simulink model "LQR_discrete"  (R2022a)
settings: Solver=VariableStepAuto  StartTime=0.0  StopTime=T_sim  RelTol=1e-3
values from neighbouring files (symbols this model uses):
  A = [-1.2822  0      0.98     0 ... (first row only)    [main.m]    (also in main_cessna.m = [-1.2822 0 0.98 0)
  B = [-0.3 ... (first row only)    [main.m]    (also in main_cessna.m)
  C = [0       1      0  0 ... (first row only)    [main.m]    (also in main_cessna.m = [0 1 0 0)
  C_states = eye(length(A))    [main.m]    (also in main_cessna.m = eye(4))
  D_states = zeros(length(B), 1)    [main.m]
  k_LQ = k_LQ4    [main.m]
  sysd = c2d(sys,T_sampling)    [main.m]
  T_sampling = 2*pi/omega_sampling    [main.m]
  u_max = deg2rad(15)    [main.m]
  u_min = deg2rad(-15)    [main.m]
  x0 = [deg2rad(0) deg2rad(15) 0 -300]    [main.m]    (also in main_cessna.m = [0 0 0 5000])
  x_ref = [0 0 0 0]    [main.m]
undefined symbols (not defined in the file or in its folder): k_LQ_d
settings Model: Creator=PaoloA  LastModifiedBy=g_mor
settings DebuggingCC: UnconnectedInputMsg=warning  UnconnectedOutputMsg=warning  UnconnectedLineMsg=warning
settings RTWCC: DLArmComputeVersion=19.05

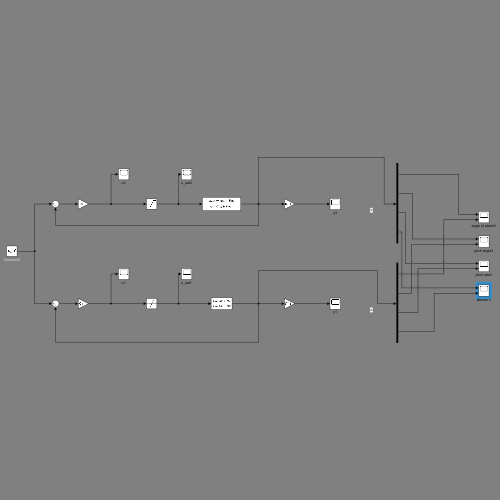
[thumbnail: Simulink's stored preview of the top-level diagram]
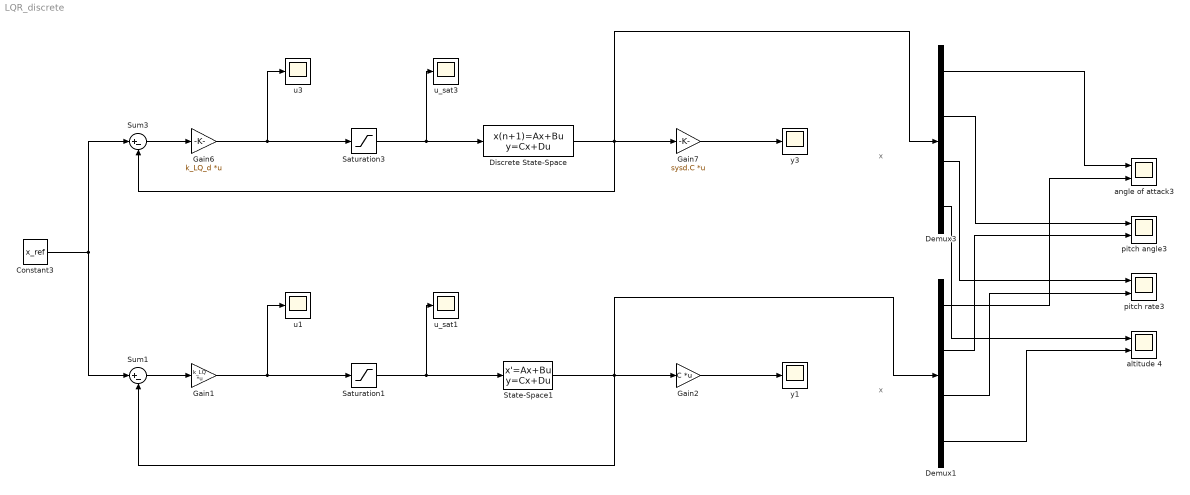
== system LQR_discrete ==
  note: x
  note: x
  Constant3 : Constant  Value=x_ref
  Demux1 : Demux
  Demux3 : Demux
  Discrete State-Space : DiscreteStateSpace  A=sysd.A  B=sysd.B  C=C_states  D=D_states  InitialCondition=x0  SampleTime=T_sampling
  Gain1 : Gain  Gain=k_LQ  Multiplication=Matrix(K*u)
  Gain2 : Gain  Gain=C  Multiplication=Matrix(K*u)
  Gain6 : Gain  Gain=k_LQ_d  Multiplication=Matrix(K*u)
  Gain7 : Gain  Gain=sysd.C  Multiplication=Matrix(K*u)
  Saturation1 : Saturate  UpperLimit=u_max  LowerLimit=u_min
  Saturation3 : Saturate  UpperLimit=u_max  LowerLimit=u_min
  State-Space1 : StateSpace  A=A  B=B  C=C_states  D=D_states  InitialCondition=x0
  Sum1 : Sum  Inputs=|+-
  Sum3 : Sum  Inputs=|+-
  altitude 4 : Scope  NumInputPorts=2
  angle of attack3 : Scope  NumInputPorts=2
  pitch angle3 : Scope  NumInputPorts=2
  pitch rate3 : Scope  NumInputPorts=2
  u1 : Scope
  u3 : Scope
  u_sat1 : Scope
  u_sat3 : Scope
  y1 : Scope
  y3 : Scope
  wires:
  Gain6/1 -> u3/1, Saturation3/1
  Constant3/1 -> Sum1/1, Sum3/1
  Sum3/1 -> Gain6/1
  Saturation3/1 -> Discrete State-Space/1, u_sat3/1
  Demux3/2 -> pitch angle3/1
  Demux3/1 -> angle of attack3/1
  Demux3/3 -> pitch rate3/1
  Demux3/4 -> altitude 4/1
  Gain7/1 -> y3/1
  Gain2/1 -> y1/1
  Gain1/1 -> u1/1, Saturation1/1
  State-Space1/1 -> Sum1/2, Demux1/1, Gain2/1
  Saturation1/1 -> u_sat1/1, State-Space1/1
  Sum1/1 -> Gain1/1
  Discrete State-Space/1 -> Sum3/2, Demux3/1, Gain7/1
  Demux1/1 -> angle of attack3/2
  Demux1/2 -> pitch angle3/2
  Demux1/3 -> pitch rate3/2
  Demux1/4 -> altitude 4/2
